simulink model "Grid_AC_PLL_22a"  (R2022a)
settings: Solver=ode23t  StartTime=0.0  StopTime=Setpoint.PLL.Tsim  RelTol=1e-3
undefined symbols (not defined in the file or in its folder): Electric, Generator, Plate, R_h2
libraries: fl_lib x32, nesl_utility x17, ee_lib x16, spsRMSLib x1, spspowerguiLib x1
(part 4 of 4)

== matlab function Grid_AC_PLL_22a/GRID/Uref calculation ==
  data: w_t input; u input; y output
function y = fcn(w_t, u)

ya = u*sin(w_t+0);
yb = u*sin(w_t-2*pi/3);
yc = u*sin(w_t+2*pi/3);

y = [ya yb yc]';

== matlab function Grid_AC_PLL_22a/Electrolyzer/Sensor/MATLAB Function ==
  data: u input; Z output
function Z = fcn(u)

Z = min(u(2)/u(1),1e3);
